simulink model "swingup_sim_19"  (R2019b)
settings: Solver=FixedStepAuto  StartTime=0.0  StopTime=30  RelTol=1e-3
values from neighbouring files (symbols this model uses):
  g = th(8,1)    [NL_eqns_Disturbance.m]    (also in NL_eqns_EKF.m; StateFcn.m; computeFJacobian.m)
  J_a = th(3,1)    [NL_eqns_Disturbance.m]    (also in NL_eqns_EKF.m; StateFcn.m; computeFJacobian.m)
  K_g = th(9,1)    [NL_eqns_Disturbance.m]    (also in NL_eqns_EKF.m; StateFcn.m; computeFJacobian.m)
  k_m = th(13,1)    [NL_eqns_Disturbance.m]    (also in NL_eqns_EKF.m; StateFcn.m; computeFJacobian.m)
  l_p = th(5,1)    [NL_eqns_Disturbance.m]    (also in NL_eqns_EKF.m; StateFcn.m; computeFJacobian.m)
  m_p = th(6,1)    [NL_eqns_Disturbance.m]    (also in NL_eqns_EKF.m; StateFcn.m; computeFJacobian.m)
  r = th(7,1)    [NL_eqns_Disturbance.m]    (also in NL_eqns_EKF.m; StateFcn.m; computeFJacobian.m)
  Ts = 0.002    [StateFcn.m]
undefined symbols (not defined in the file or in its folder): A_ob, B_ob, c1_tau, C_ob, D_ob, DiscIntNeverNeededParam, E, id_param, Jp_prime, Kd, Kp, Kpp, P0, R, voltage_max, x0_down, x0_KF, x0_ob
libraries: sharedTrackingLibrary x1
settings Model: Creator=federicocorso  LastModifiedBy=federicocorso
settings DebuggingCC: UnconnectedInputMsg=none  UnconnectedOutputMsg=none  UnconnectedLineMsg=none  SFMachineParentedDataDiag=error
settings ModelReferenceCC: EnableRefExpFcnMdlSchedulingChecks=off
settings RTWCC: Description=Generic Real-Time Target  GenCodeOnly=on

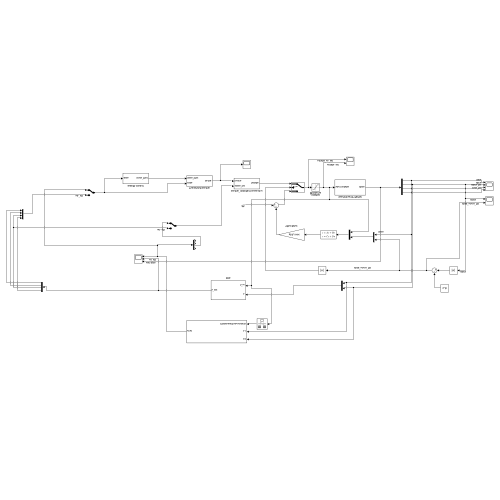
[thumbnail: Simulink's stored preview of the top-level diagram]
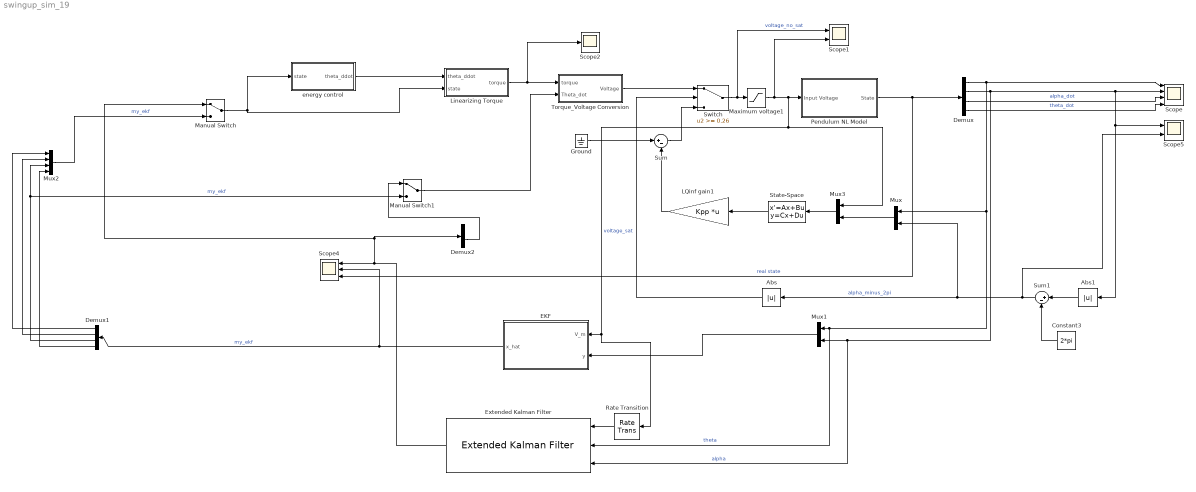
== system swingup_sim_19 ==
  Abs : Abs
  Abs1 : Abs
  Constant3 : Constant  Value=2*pi
  Demux : Demux
  Demux1 : Demux
  Demux2 : Demux
  EKF : Subsystem
  Extended Kalman Filter : sharedTrackingLibrary/Extended Kalman Filter  StateTransitionFcn=StateFcn  HasStateTransitionJacobianFcn=off  HasAdditiveProcessNoise=Additive  ProcessNoise=0  HasTimeVaryingProcessNoise=off  HasStateTransitionFcnExtraArgument=1  InitialState=x0_KF  InitialStateCovariance=P0  MeasurementFcn1=measurementFcn1  HasMeasurementJacobianFcn1=off  HasMeasurementEnablePort1=off  HasAdditiveMeasurementNoise1=Additive  MeasurementNoise1=rho_theta_meas  HasTimeVaryingMeasurementNoise1=off  HasMeasurementFcnExtraArgument1=0  HasMeasurementWrapping1=off  MeasurementFcn2=measurementFcn2  HasMeasurementJacobianFcn2=off  HasMeasurementEnablePort2=off  HasAdditiveMeasurementNoise2=Additive  MeasurementNoise2=rho_alpha_meas  HasTimeVaryingMeasurementNoise2=off  HasMeasurementFcnExtraArgument2=0  HasMeasurementWrapping2=off  MeasurementFcn3=myMeasurementFcn  HasMeasurementJacobianFcn3=off  HasMeasurementEnablePort3=off  HasAdditiveMeasurementNoise3=Additive  MeasurementNoise3=1  HasTimeVaryingMeasurementNoise3=off  HasMeasurementFcnExtraArgument3=0  HasMeasurementWrapping3=off  MeasurementFcn4=myMeasurementFcn  HasMeasurementJacobianFcn4=off  HasMeasurementEnablePort4=off  HasAdditiveMeasurementNoise4=Additive  MeasurementNoise4=1  HasTimeVaryingMeasurementNoise4=off  HasMeasurementFcnExtraArgument4=0  HasMeasurementWrapping4=off  MeasurementFcn5=myMeasurementFcn  HasMeasurementJacobianFcn5=off  HasMeasurementEnablePort5=off  HasAdditiveMeasurementNoise5=Additive  MeasurementNoise5=1  HasTimeVaryingMeasurementNoise5=off  HasMeasurementFcnExtraArgument5=0  HasMeasurementWrapping5=off  EnableMultirate=off  StateTransitionFcnSampleTime=1  MeasurementFcn1SampleTime=1  MeasurementFcn2SampleTime=1  MeasurementFcn3SampleTime=1  MeasurementFcn4SampleTime=1  MeasurementFcn5SampleTime=1  UseCurrentEstimator=on  OutputStateCovariance=off  DataType=double  SampleTime=Ts  NumberOfMeasurements=2
  Ground : Ground
  LQinf gain1 : Gain  Gain=Kpp  Multiplication=Matrix(K*u) (u vector)
  Linearizing Torque : Subsystem
  Manual Switch : ManualSwitch
  Manual Switch1 : ManualSwitch
  Maximum voltage1 : Saturate  UpperLimit=voltage_max  LowerLimit=-voltage_max
  Mux : Mux  Inputs=2
  Mux1 : Mux  Inputs=2
  Mux2 : Mux
  Mux3 : Mux  Inputs=2
  Pendulum NL Model : Subsystem
  Rate Transition : RateTransition
  Scope : Scope  NumInputPorts=4
  Scope1 : Scope  NumInputPorts=2
  Scope2 : Scope
  Scope4 : Scope  NumInputPorts=3
  Scope5 : Scope  NumInputPorts=2
  State-Space : StateSpace  A=A_ob  B=B_ob  C=C_ob  D=D_ob  InitialCondition=x0_ob
  Sum : Sum  Inputs=|+-
  Sum1 : Sum  Inputs=|+-
  Switch : Switch  Threshold=0.26
  Torque_Voltage Conversion : Subsystem
  energy control : Subsystem
  wires:
  Linearizing Torque/1(torque) -> Torque_Voltage Conversion/1(torque), Scope2/1
  Demux/1 -> Mux/1, Extended Kalman Filter/2, Mux1/1, Scope/1  "theta"
  Demux/3 -> Scope/3  "alpha_dot"
  Demux/4 -> Scope/4  "theta_dot"
  Demux1/3 -> Manual Switch1/2, Mux2/3  "my_ekf"
  energy control/1(theta_ddot) -> Linearizing Torque/1(theta_ddot)
  Demux/2 -> Mux1/2, Extended Kalman Filter/3, Scope5/1, Abs1/1, Scope/2  "alpha"
  LQinf gain1/1 -> Sum/2
  Ground/1 -> Sum/1
  Pendulum NL Model/1(State) -> Scope4/3, Demux/1  "real state"
  Mux1/1 -> EKF/2(y)
  EKF/1(x_hat) -> Demux1/1, Scope4/2  "my_ekf"
  Demux1/4 -> Mux2/4
  Demux1/2 -> Mux2/2
  Demux1/1 -> Mux2/1
  Sum/1 -> Switch/3
  Torque_Voltage Conversion/1(Voltage) -> Switch/1
  Mux2/1 -> Manual Switch/2  "my_ekf"
  Switch/1 -> Scope1/1, Maximum voltage1/1  "voltage_no_sat"
  Mux/1 -> Mux3/2
  Abs/1 -> Switch/2
  Abs1/1 -> Sum1/1
  Constant3/1 -> Sum1/2
  Sum1/1 -> Abs/1, Mux/2, Scope5/2  "alpha_minus_2pi"
  State-Space/1 -> LQinf gain1/1
  Mux3/1 -> State-Space/1
  Maximum voltage1/1 -> Scope1/2, Rate Transition/1, EKF/1(V_m), Mux3/1, Pendulum NL Model/1(Input Voltage)  "voltage_sat"
  Manual Switch/1 -> energy control/1(state), Linearizing Torque/2(state)
  Manual Switch1/1 -> Torque_Voltage Conversion/2(Theta_dot)
  Extended Kalman Filter/1 -> Manual Switch/1, Demux2/1, Scope4/1
  Rate Transition/1 -> Extended Kalman Filter/1
  Demux2/3 -> Manual Switch1/1

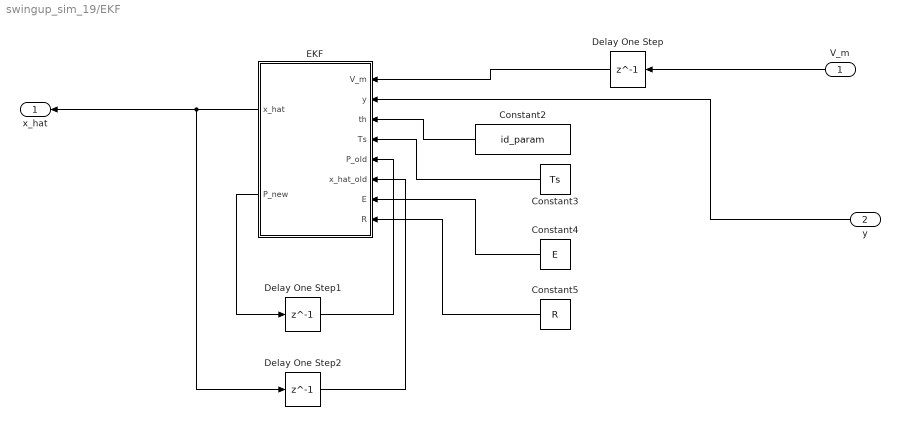
== system swingup_sim_19/EKF ==
  V_m : Inport
  y : Inport  Port=2
  Constant2 : Constant  Value=id_param
  Constant3 : Constant  Value=Ts
  Constant4 : Constant  Value=E
  Constant5 : Constant  Value=R
  Delay One Step : Delay  DelayLength=1
  Delay One Step1 : Delay  DelayLength=1  InitialCondition=P0  SampleTime=Ts
  Delay One Step2 : Delay  DelayLength=1  InitialCondition=x0_KF  SampleTime=Ts
  EKF : MATLAB Function  TreatAsAtomicUnit=on
  x_hat : Outport
  wires:
  Constant5/1 -> EKF/8(R)
  y/1 -> EKF/2(y)
  Constant2/1 -> EKF/3(th)
  EKF/1(x_hat) -> Delay One Step2/1, x_hat/1
  V_m/1 -> Delay One Step/1
  Constant3/1 -> EKF/4(Ts)
  Constant4/1 -> EKF/7(E)
  EKF/2(P_new) -> Delay One Step1/1
  Delay One Step1/1 -> EKF/5(P_old)
  Delay One Step2/1 -> EKF/6(x_hat_old)
  Delay One Step/1 -> EKF/1(V_m)

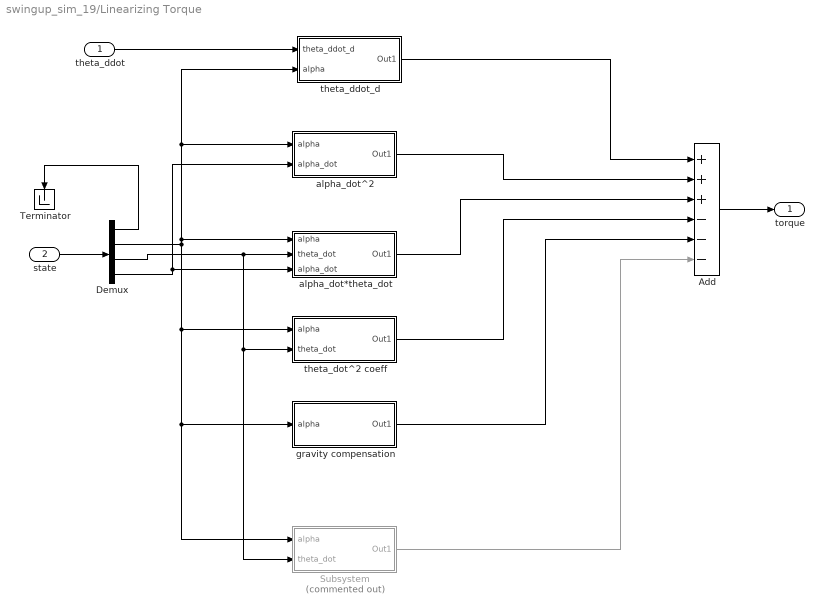
== system swingup_sim_19/Linearizing Torque ==
  theta_ddot : Inport
  state : Inport  Port=2
  Add : Sum  Inputs=+++---
  Demux : Demux
  Subsystem : Subsystem  Commented=on
  Terminator : Terminator
  alpha_dot*theta_dot : Subsystem
  alpha_dot^2 : Subsystem
  gravity compensation : Subsystem
  theta_ddot_d : Subsystem
  theta_dot^2 coeff : Subsystem
  torque : Outport
  wires:
  Add/1 -> torque/1
  gravity compensation/1(Out1) -> Add/5
  theta_dot^2 coeff/1(Out1) -> Add/4
  alpha_dot*theta_dot/1(Out1) -> Add/3
  alpha_dot^2/1(Out1) -> Add/2
  theta_ddot_d/1(Out1) -> Add/1
  theta_ddot/1 -> theta_ddot_d/1(theta_ddot_d)
  state/1 -> Demux/1
  Demux/1 -> Terminator/1
  Demux/2 -> Subsystem/1(alpha), gravity compensation/1(alpha), theta_dot^2 coeff/1(alpha), alpha_dot*theta_dot/1(alpha), alpha_dot^2/1(alpha), theta_ddot_d/2(alpha)
  Demux/3 -> theta_dot^2 coeff/2(theta_dot), Subsystem/2(theta_dot), alpha_dot*theta_dot/2(theta_dot)
  Demux/4 -> alpha_dot*theta_dot/3(alpha_dot), alpha_dot^2/2(alpha_dot)
  Subsystem/1(Out1) -> Add/6

== system swingup_sim_19/Pendulum NL Model ==
  Input Voltage : Inport
  Constant : Constant  Value=id_param
  Discrete-Time Integrator : DiscreteIntegrator  InitialCondition=x0_down  SampleTime=Ts  ICPrevOutput=DiscIntNeverNeededParam  ICPrevScaledInput=DiscIntNeverNeededParam
  MATLAB Function : MATLAB Function  TreatAsAtomicUnit=on
  State : Outport
  wires:
  Input Voltage/1 -> MATLAB Function/2(V_m)
  Constant/1 -> MATLAB Function/3(th)
  MATLAB Function/1(x_dot) -> Discrete-Time Integrator/1
  Discrete-Time Integrator/1 -> State/1, MATLAB Function/1(x)

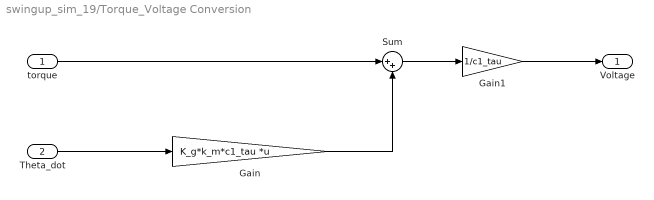
== system swingup_sim_19/Torque_Voltage Conversion ==
  torque : Inport
  Theta_dot : Inport  Port=2
  Gain : Gain  Gain=K_g*k_m*c1_tau  Multiplication=Matrix(K*u)
  Gain1 : Gain  Gain=1/c1_tau
  Sum : Sum  Inputs=|++
  Voltage : Outport
  wires:
  Theta_dot/1 -> Gain/1
  Gain1/1 -> Voltage/1
  Sum/1 -> Gain1/1
  Gain/1 -> Sum/2
  torque/1 -> Sum/1

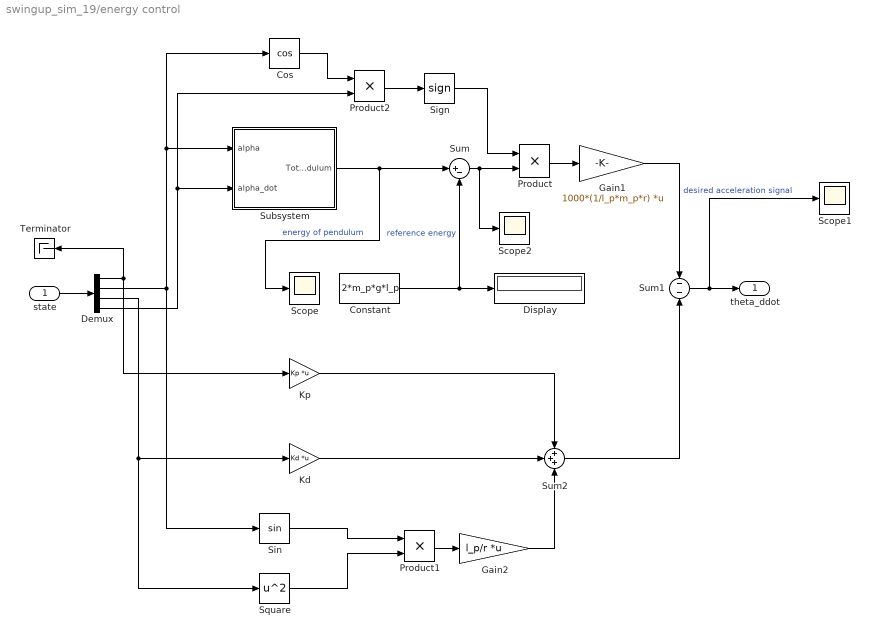
== system swingup_sim_19/energy control ==
  state : Inport
  Constant : Constant  Value=2*m_p*g*l_p
  Cos : Trigonometry  Operator=cos
  Demux : Demux
  Display : Display
  Gain1 : Gain  Gain=1000*(1/l_p*m_p*r)  Multiplication=Matrix(K*u)
  Gain2 : Gain  Gain=l_p/r  Multiplication=Matrix(K*u)
  Kd : Gain  Gain=Kd  Multiplication=Matrix(K*u)
  Kp : Gain  Gain=Kp  Multiplication=Matrix(K*u)
  Product : Product
  Product1 : Product
  Product2 : Product
  Scope : Scope
  Scope1 : Scope
  Scope2 : Scope
  Sign : Signum
  Sin : Trigonometry
  Square : Math  Operator=square  SaturateOnIntegerOverflow=on
  Subsystem : Subsystem
  Sum : Sum  Inputs=|+-
  Sum1 : Sum  Inputs=--
  Sum2 : Sum  Inputs=+++
  Terminator : Terminator
  theta_ddot : Outport
  wires:
  state/1 -> Demux/1
  Demux/2 -> Sin/1, Subsystem/1(alpha), Cos/1
  Demux/4 -> Subsystem/2(alpha_dot), Product2/2
  Cos/1 -> Product2/1
  Product/1 -> Gain1/1
  Gain2/1 -> Sum2/3
  Product1/1 -> Gain2/1
  Demux/3 -> Square/1, Kd/1
  Demux/1 -> Kp/1, Terminator/1
  Sin/1 -> Product1/1
  Square/1 -> Product1/2
  Product2/1 -> Sign/1
  Subsystem/1(Total Energy Pendulum) -> Sum/1, Scope/1  "energy of pendulum"
  Sum1/1 -> Scope1/1, theta_ddot/1  "desired acceleration signal"
  Kp/1 -> Sum2/1
  Kd/1 -> Sum2/2
  Sum2/1 -> Sum1/2
  Gain1/1 -> Sum1/1
  Sum/1 -> Scope2/1, Product/2
  Constant/1 -> Display/1, Sum/2  "reference energy"
  Sign/1 -> Product/1

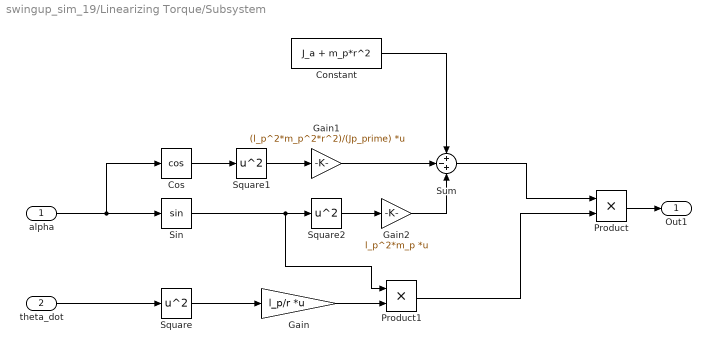
== system swingup_sim_19/Linearizing Torque/Subsystem ==
  alpha : Inport
  theta_dot : Inport  Port=2
  Constant : Constant  Value=J_a + m_p*r^2
  Cos : Trigonometry  Operator=cos
  Gain : Gain  Gain=l_p/r  Multiplication=Matrix(K*u)
  Gain1 : Gain  Gain=(l_p^2*m_p^2*r^2)/(Jp_prime)  Multiplication=Matrix(K*u)
  Gain2 : Gain  Gain=l_p^2*m_p  Multiplication=Matrix(K*u)
  Product : Product
  Product1 : Product
  Sin : Trigonometry
  Square : Math  Operator=square  SaturateOnIntegerOverflow=on
  Square1 : Math  Operator=square  SaturateOnIntegerOverflow=on
  Square2 : Math  Operator=square  SaturateOnIntegerOverflow=on
  Sum : Sum  Inputs=+-+
  Out1 : Outport
  wires:
  theta_dot/1 -> Square/1
  alpha/1 -> Sin/1, Cos/1
  Square/1 -> Gain/1
  Product/1 -> Out1/1
  Gain/1 -> Product1/2
  Sin/1 -> Square2/1, Product1/1
  Cos/1 -> Square1/1
  Square1/1 -> Gain1/1
  Gain1/1 -> Sum/2
  Square2/1 -> Gain2/1
  Gain2/1 -> Sum/3
  Constant/1 -> Sum/1
  Sum/1 -> Product/1
  Product1/1 -> Product/2

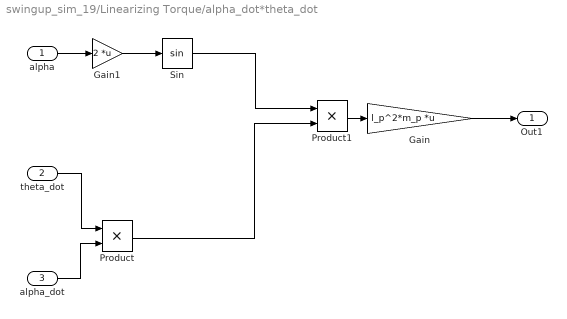
== system swingup_sim_19/Linearizing Torque/alpha_dot*theta_dot ==
  alpha : Inport
  theta_dot : Inport  Port=2
  alpha_dot : Inport  Port=3
  Gain : Gain  Gain=l_p^2*m_p  Multiplication=Matrix(K*u)
  Gain1 : Gain  Gain=2  Multiplication=Matrix(K*u)
  Product : Product
  Product1 : Product
  Sin : Trigonometry
  Out1 : Outport
  wires:
  theta_dot/1 -> Product/1
  alpha_dot/1 -> Product/2
  Gain/1 -> Out1/1
  Product1/1 -> Gain/1
  Product/1 -> Product1/2
  alpha/1 -> Gain1/1
  Gain1/1 -> Sin/1
  Sin/1 -> Product1/1

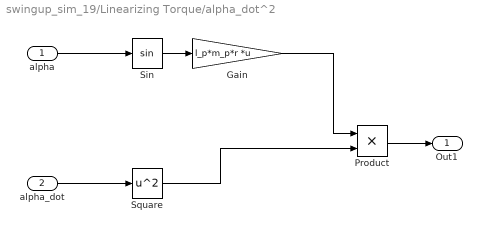
== system swingup_sim_19/Linearizing Torque/alpha_dot^2 ==
  alpha : Inport
  alpha_dot : Inport  Port=2
  Gain : Gain  Gain=l_p*m_p*r  Multiplication=Matrix(K*u)
  Product : Product
  Sin : Trigonometry
  Square : Math  Operator=square  SaturateOnIntegerOverflow=on
  Out1 : Outport
  wires:
  alpha_dot/1 -> Square/1
  Product/1 -> Out1/1
  Square/1 -> Product/2
  alpha/1 -> Sin/1
  Sin/1 -> Gain/1
  Gain/1 -> Product/1

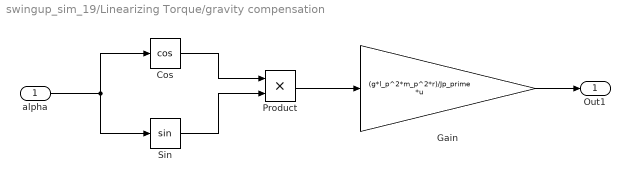
== system swingup_sim_19/Linearizing Torque/gravity compensation ==
  alpha : Inport
  Cos : Trigonometry  Operator=cos
  Gain : Gain  Gain=(g*l_p^2*m_p^2*r)/Jp_prime  Multiplication=Matrix(K*u)
  Product : Product
  Sin : Trigonometry
  Out1 : Outport
  wires:
  Gain/1 -> Out1/1
  Product/1 -> Gain/1
  Cos/1 -> Product/1
  Sin/1 -> Product/2
  alpha/1 -> Cos/1, Sin/1

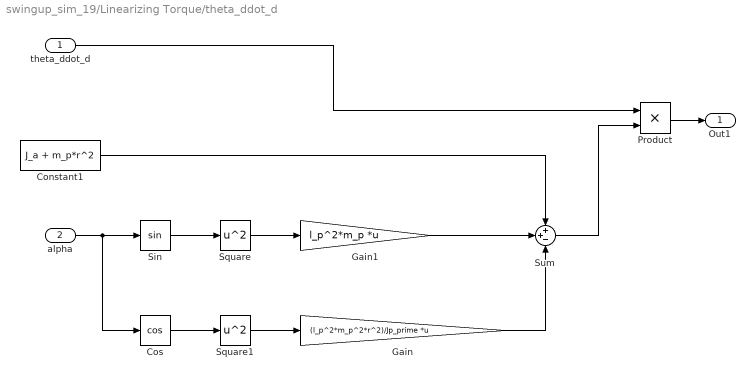
== system swingup_sim_19/Linearizing Torque/theta_ddot_d ==
  theta_ddot_d : Inport
  alpha : Inport  Port=2
  Constant1 : Constant  Value=J_a + m_p*r^2
  Cos : Trigonometry  Operator=cos
  Gain : Gain  Gain=(l_p^2*m_p^2*r^2)/Jp_prime  Multiplication=Matrix(K*u)
  Gain1 : Gain  Gain=l_p^2*m_p  Multiplication=Matrix(K*u)
  Product : Product
  Sin : Trigonometry
  Square : Math  Operator=square  SaturateOnIntegerOverflow=on
  Square1 : Math  Operator=square  SaturateOnIntegerOverflow=on
  Sum : Sum  Inputs=++-
  Out1 : Outport
  wires:
  Product/1 -> Out1/1
  theta_ddot_d/1 -> Product/1
  Sin/1 -> Square/1
  alpha/1 -> Sin/1, Cos/1
  Cos/1 -> Square1/1
  Square/1 -> Gain1/1
  Square1/1 -> Gain/1
  Constant1/1 -> Sum/1
  Gain1/1 -> Sum/2
  Gain/1 -> Sum/3
  Sum/1 -> Product/2

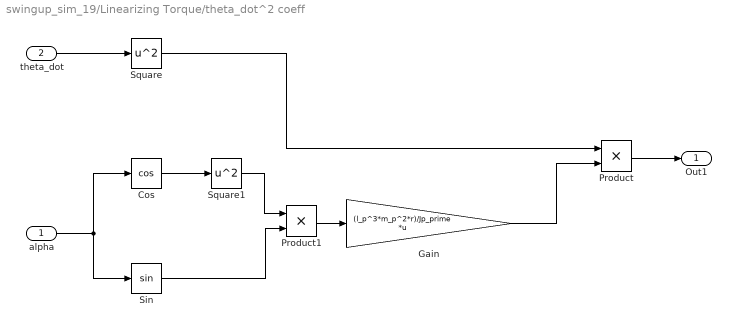
== system swingup_sim_19/Linearizing Torque/theta_dot^2 coeff ==
  alpha : Inport
  theta_dot : Inport  Port=2
  Cos : Trigonometry  Operator=cos
  Gain : Gain  Gain=(l_p^3*m_p^2*r)/Jp_prime  Multiplication=Matrix(K*u)
  Product : Product
  Product1 : Product
  Sin : Trigonometry
  Square : Math  Operator=square  SaturateOnIntegerOverflow=on
  Square1 : Math  Operator=square  SaturateOnIntegerOverflow=on
  Out1 : Outport
  wires:
  theta_dot/1 -> Square/1
  Product/1 -> Out1/1
  Square/1 -> Product/1
  Cos/1 -> Square1/1
  alpha/1 -> Sin/1, Cos/1
  Product1/1 -> Gain/1
  Square1/1 -> Product1/1
  Sin/1 -> Product1/2
  Gain/1 -> Product/2

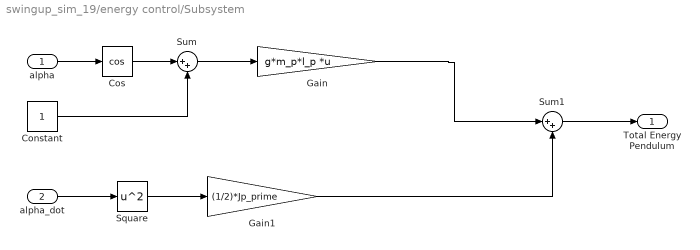
== system swingup_sim_19/energy control/Subsystem ==
  alpha : Inport
  alpha_dot : Inport  Port=2
  Constant : Constant
  Cos : Trigonometry  Operator=cos
  Gain : Gain  Gain=g*m_p*l_p  Multiplication=Matrix(K*u)
  Gain1 : Gain  Gain=(1/2)*Jp_prime
  Square : Math  Operator=square  SaturateOnIntegerOverflow=on
  Sum : Sum  Inputs=|++
  Sum1 : Sum  Inputs=|++
  Total Energy Pendulum : Outport
  wires:
  alpha/1 -> Cos/1
  Cos/1 -> Sum/1
  Constant/1 -> Sum/2
  Sum/1 -> Gain/1
  Sum1/1 -> Total Energy Pendulum/1
  Gain/1 -> Sum1/1
  alpha_dot/1 -> Square/1
  Square/1 -> Gain1/1
  Gain1/1 -> Sum1/2

== matlab function swingup_sim_19/EKF/EKF ==
  data: V_m input; x_hat output; y input; th input; Ts input; P_old input; x_hat_old input; E input; R input; P_new output
function [x_hat,P_new] = fcn(V_m,y,th,Ts,P_old,x_hat_old,E,R)
% INPUTS
% V_m: input variable, the voltage
% y: measured state
% th: vector of dynamical parameters of the pendulum
% Ts: sampling time for the DT model used in the filter
% P_old: previous state covariance matrix
% x_hat_old: previous state 
% E process covariance matrix
% R measurement covariance matrix

%% Physical params
B_p = th(1,1);
B_r = th(2,1);
J_a = th(3,1);
J_p = th(4,1);
l_p = th(5,1);
m_p = th(6,1);
r = th(7,1);
g = th(8,1);
K_g = th(9,1);
R_m = th(10,1);
eta_g = th(11,1);
eta_m = th(12,1);
k_m = th(13,1);
k_t = th(14,1);

%% computing state derivative of non linear model
tau = eta_g*K_g*eta_m*k_t*(V_m-K_g*k_m*x_hat_old(3,1))/R_m; % motor torque expression-STATIC

t2 = cos(x_hat_old(2,1));
t3 = sin(x_hat_old(2,1));
t4 = l_p.^2;
t5 = l_p.^3;
t7 = m_p.^2;
t8 = r.^2;
t9 = x_hat_old(2,1).*2.0;
t10 = x_hat_old(3,1).^2;
t11 = x_hat_old(4,1).^2;
t12 = J_a.*J_p;
t6 = t4.^2;
t13 = t2.^2;
t14 = sin(t9);
t15 = J_a.*m_p.*t4;
t16 = J_p.*m_p.*t4;
t17 = J_p.*m_p.*t8;
t20 = t4.*t7.*t8;
t18 = t6.*t7;
t19 = t13.*t16;
t24 = t13.*t20;
t21 = t13.*t18;
t22 = -t19;
t25 = -t24;
t23 = -t21;
t26 = t12+t15+t16+t17+t18+t20+t22+t23+t25;
t27 = 1.0./t26;

x_dot = zeros(4,1);

x_dot(1,1) = x_hat_old(3,1);
x_dot(2,1) = x_hat_old(4,1);
x_dot(3,1) = t27.*(J_p.*tau.*-2.0+B_r.*J_p.*x_hat_old(3,1).*2.0-m_p.*t4.*tau.*2.0+t14.*t16.*x_hat_old(3,1).*x_hat_old(4,1).*2.0+t14.*t18.*x_hat_old(3,1).*x_hat_old(4,1).*2.0+B_r.*m_p.*t4.*x_hat_old(3,1).*2.0+r.*t3.*t5.*t7.*t11.*2.0-g.*r.*t2.*t3.*t4.*t7.*2.0-r.*t2.*t5.*t7.*t10.*t14+B_p.*l_p.*m_p.*r.*t2.*x_hat_old(4,1).*2.0+J_p.*l_p.*m_p.*r.*t3.*t11.*2.0).*(-1.0./2.0);
x_dot(4,1) = t27.*(B_p.*J_a.*x_hat_old(4,1).*2.0-t10.*t14.*t15-t10.*t14.*t18-t10.*t14.*t20+t10.*t14.*t21-g.*t3.*t5.*t7.*2.0+t2.*t3.*t11.*t20.*2.0+B_p.*m_p.*t4.*x_hat_old(4,1).*2.0+B_p.*m_p.*t8.*x_hat_old(4,1).*2.0-J_a.*g.*l_p.*m_p.*t3.*2.0-B_p.*m_p.*t4.*t13.*x_hat_old(4,1).*2.0-g.*l_p.*t3.*t7.*t8.*2.0-l_p.*m_p.*r.*t2.*tau.*2.0+g.*t3.*t5.*t7.*t13.*2.0+B_r.*l_p.*m_p.*r.*t2.*x_hat_old(3,1).*2.0+r.*t2.*t5.*t7.*t14.*x_hat_old(3,1).*x_hat_old(4,1).*2.0).*(-1.0./2.0);

%% %{=============== PREDICTION =============}%
x = x_hat_old + Ts*x_dot; % FW Euler simulation one step ahead
%% computing the local jacobian
t2 = cos(x(2));
t3 = sin(x(2));
t4 = K_g.^2;
t5 = l_p.^2;
t6 = l_p.^3;
t8 = m_p.^2;
t9 = r.^2;
t10 = x(2).*2.0;
t11 = x(2).*3.0;
t12 = x(3).^2;
t13 = x(4).^2;
t14 = J_a.*J_p;
t20 = 1.0./R_m;
t7 = t5.^2;
t15 = cos(t10);
t16 = cos(t11);
t17 = t2.^2;
t18 = sin(t10);
t19 = t3.^2;
t21 = m_p.*t5;
t22 = m_p.*t9;
t29 = t5.*t8.*t9;
t23 = J_a.*t21;
t24 = J_p.*t21;
t25 = J_p.*t22;
t26 = t19-1.0;
t27 = t7.*t8;
t32 = J_p+t21+t22;
t34 = t17.*t29;
t28 = t17.*t24;
t30 = t17.*t27;
t35 = -t34;
t31 = -t28;
t33 = -t30;
t36 = t14+t23+t24+t25+t27+t29+t31+t33+t35;
t37 = 1.0./t36;
t38 = t37.^2;
et1 = -(Ts.*l_p.*m_p.*(J_p.*r.*t2.*t13.*4.0-r.*t2.*t12.*t21+r.*t2.*t13.*t21.*4.0-r.*t12.*t16.*t21.*3.0-B_p.*r.*t3.*x(4).*4.0+J_p.*l_p.*t15.*x(3).*x(4).*8.0-g.*l_p.*m_p.*r.*t15.*4.0+m_p.*t6.*t15.*x(3).*x(4).*8.0))./(t14.*4.0+t23.*4.0+t24.*2.0+t25.*4.0+t27.*2.0+t29.*2.0-t15.*t24.*2.0-t15.*t27.*2.0-t15.*t29.*2.0);
et2 = (Ts.*t18.*t21.*t32.*t38.*(B_r.*J_p.*x(3).*2.0+B_r.*t21.*x(3).*2.0+t18.*t24.*x(3).*x(4).*2.0+t18.*t27.*x(3).*x(4).*2.0-g.*r.*t5.*t8.*t18+r.*t3.*t6.*t8.*t13.*2.0+r.*t3.*t6.*t8.*t12.*t26.*2.0+B_p.*l_p.*m_p.*r.*t2.*x(4).*2.0+J_p.*l_p.*m_p.*r.*t3.*t13.*2.0-K_g.*V_m.*eta_g.*eta_m.*k_t.*t20.*t21.*2.0-J_p.*K_g.*V_m.*eta_g.*eta_m.*k_t.*t20.*2.0+J_p.*eta_g.*eta_m.*k_m.*k_t.*t4.*t20.*x(3).*2.0+eta_g.*eta_m.*k_m.*k_t.*t4.*t20.*t21.*x(3).*2.0))./2.0;
et3 = (Ts.*l_p.*m_p.*t20.*(R_m.*g.*t2.*t21.*3.0+R_m.*g.*t2.*t22.*4.0-R_m.*g.*t16.*t21.*3.0+J_a.*R_m.*g.*t2.*4.0-R_m.*m_p.*t6.*t12.*cos(x(2).*4.0).*2.0-B_p.*R_m.*l_p.*t18.*x(4).*4.0+J_a.*R_m.*l_p.*t12.*t15.*4.0+B_r.*R_m.*r.*t3.*x(3).*4.0+R_m.*l_p.*t12.*t15.*t22.*4.0-R_m.*l_p.*t13.*t15.*t22.*4.0+R_m.*m_p.*t6.*t12.*t15.*2.0-R_m.*r.*t2.*t21.*x(3).*x(4).*2.0-R_m.*r.*t16.*t21.*x(3).*x(4).*6.0-K_g.*V_m.*eta_g.*eta_m.*k_t.*r.*t3.*4.0+eta_g.*eta_m.*k_m.*k_t.*r.*t3.*t4.*x(3).*4.0))./(t14.*4.0+t23.*4.0+t24.*2.0+t25.*4.0+t27.*2.0+t29.*2.0-t15.*t24.*2.0-t15.*t27.*2.0-t15.*t29.*2.0);
et4 = Ts.*t18.*t21.*t32.*t38.*(B_p.*J_a.*x(4).*-2.0-B_p.*t21.*x(4).*2.0-B_p.*t22.*x(4).*2.0+t12.*t18.*t23+t12.*t18.*t27+t12.*t18.*t29-t13.*t18.*t29+B_p.*t17.*t21.*x(4).*2.0+g.*t3.*t6.*t8.*2.0-t2.^3.*t3.*t12.*t27.*2.0-g.*t6.*t8.*(t3-t3.^3).*2.0+J_a.*g.*l_p.*m_p.*t3.*2.0+g.*l_p.*t3.*t8.*t9.*2.0-B_r.*l_p.*m_p.*r.*t2.*x(3).*2.0+r.*t3.*t6.*t8.*t26.*x(3).*x(4).*4.0+K_g.*eta_g.*eta_m.*k_t.*l_p.*m_p.*r.*t2.*t20.*(V_m-K_g.*k_m.*x(3)).*2.0).*(-1.0./2.0);
mt1 = [1.0,0.0,0.0,0.0,0.0,1.0,et1+et2,et3+et4,Ts,0.0,Ts.*t37.*(B_r.*t21.*2.0+B_r.*J_p.*2.0+t18.*t24.*x(4).*2.0+t18.*t27.*x(4).*2.0-r.*t2.*t6.*t8.*t18.*x(3).*2.0+J_p.*eta_g.*eta_m.*k_m.*k_t.*t4.*t20.*2.0+eta_g.*eta_m.*k_m.*k_t.*t4.*t20.*t21.*2.0).*(-1.0./2.0)+1.0,Ts.*t37.*(t18.*t23.*x(3).*-2.0-t18.*t27.*x(3).*2.0-t18.*t29.*x(3).*2.0+t18.*t30.*x(3).*2.0+B_r.*l_p.*m_p.*r.*t2.*2.0+r.*t2.*t6.*t8.*t18.*x(4).*2.0+eta_g.*eta_m.*k_m.*k_t.*l_p.*m_p.*r.*t2.*t4.*t20.*2.0).*(-1.0./2.0),0.0,Ts,-Ts.*l_p.*m_p.*t37.*(B_p.*r.*t2+J_p.*l_p.*t18.*x(3)+J_p.*r.*t3.*x(4).*2.0+m_p.*t6.*t18.*x(3)+r.*t3.*t21.*x(4).*2.0)];
mt2 = [Ts.*t37.*(B_p.*t21.*2.0+B_p.*t22.*2.0+B_p.*J_a.*2.0-B_p.*t17.*t21.*2.0+t2.*t3.*t29.*x(4).*4.0+r.*t3.*t6.*t8.*t17.*x(3).*4.0).*(-1.0./2.0)+1.0];
F_eval = reshape([mt1,mt2],4,4);

F_k = F_eval; % jacobian matrix

%% covariance and output
P_temp = F_k*P_old*(F_k') + E; % update covariance matrix
yK = [x(1);x(2)]; % compute output prediction estimate

%% %{========================================}%
%% %{=============== CORRECTION =============}%

H = eye(2,4); % output matrix
I = eye(4);
% innovation
e =  y - yK; % difference between real meas. and predicted output
Ht = H'; % H transposed, compute just once and use 2 times
S = H*P_temp*Ht + R;  % % residual covariance

% near optimal Kalman Gain
K =  (P_temp*Ht)/S;

% updated state estimate
x_hat = x + K*e; % feedback correction
% updated covariance estimate
P_new = (I-K*H)*P_temp;

== matlab function swingup_sim_19/Pendulum NL Model/MATLAB Function ==
  data: x input; x_dot output; V_m input; th input
function x_dot = NL_eqns(x,V_m,th)
%NL_eqns
%    NL_DIFF_EQNS_SS = NL_eqns(B_p,B_r,J_a,J_p,G,L_P,M_P,R,TAU,x(2,1),x(3,1),x(4,1),X_DOT_1,X_DOT_2,X_DOT_3,X_DOT_4)

%    This function was generated by the Symbolic Math Toolbox version 9.2.
%    09-Mar-2023 15:34:15
B_p = th(1,1);
B_r = th(2,1);
J_a = th(3,1);
J_p = th(4,1);
l_p = th(5,1);
m_p = th(6,1);
r = th(7,1);
g = th(8,1);
K_g = th(9,1);
R_m = th(10,1);
eta_g = th(11,1);
eta_m = th(12,1);
k_m = th(13,1);
k_t = th(14,1);

tau = eta_g*K_g*eta_m*k_t*(V_m-K_g*k_m*x(3,1))/R_m; % motor torque expression-STATIC

t2 = cos(x(2,1));
t3 = sin(x(2,1));
t4 = l_p.^2;
t5 = l_p.^3;
t7 = m_p.^2;
t8 = r.^2;
t9 = x(2,1).*2.0;
t10 = x(3,1).^2;
t11 = x(4,1).^2;
t12 = J_a.*J_p;
t6 = t4.^2;
t13 = t2.^2;
t14 = sin(t9);
t15 = J_a.*m_p.*t4;
t16 = J_p.*m_p.*t4;
t17 = J_p.*m_p.*t8;
t20 = t4.*t7.*t8;
t18 = t6.*t7;
t19 = t13.*t16;
t24 = t13.*t20;
t21 = t13.*t18;
t22 = -t19;
t25 = -t24;
t23 = -t21;
t26 = t12+t15+t16+t17+t18+t20+t22+t23+t25;
t27 = 1.0./t26;

x_dot = zeros(4,1);

x_dot(1,1) = x(3,1);
x_dot(2,1) = x(4,1);
x_dot(3,1) = t27.*(J_p.*tau.*-2.0+B_r.*J_p.*x(3,1).*2.0-m_p.*t4.*tau.*2.0+t14.*t16.*x(3,1).*x(4,1).*2.0+t14.*t18.*x(3,1).*x(4,1).*2.0+B_r.*m_p.*t4.*x(3,1).*2.0+r.*t3.*t5.*t7.*t11.*2.0-g.*r.*t2.*t3.*t4.*t7.*2.0-r.*t2.*t5.*t7.*t10.*t14+B_p.*l_p.*m_p.*r.*t2.*x(4,1).*2.0+J_p.*l_p.*m_p.*r.*t3.*t11.*2.0).*(-1.0./2.0);
x_dot(4,1) = t27.*(B_p.*J_a.*x(4,1).*2.0-t10.*t14.*t15-t10.*t14.*t18-t10.*t14.*t20+t10.*t14.*t21-g.*t3.*t5.*t7.*2.0+t2.*t3.*t11.*t20.*2.0+B_p.*m_p.*t4.*x(4,1).*2.0+B_p.*m_p.*t8.*x(4,1).*2.0-J_a.*g.*l_p.*m_p.*t3.*2.0-B_p.*m_p.*t4.*t13.*x(4,1).*2.0-g.*l_p.*t3.*t7.*t8.*2.0-l_p.*m_p.*r.*t2.*tau.*2.0+g.*t3.*t5.*t7.*t13.*2.0+B_r.*l_p.*m_p.*r.*t2.*x(3,1).*2.0+r.*t2.*t5.*t7.*t14.*x(3,1).*x(4,1).*2.0).*(-1.0./2.0);
